simulink model "get_step"  (R2020b)
settings: Solver=FixedStepAuto  StartTime=0.0  StopTime=90  MaxStep=1  RelTol=1e-3
undefined symbols (not defined in the file or in its folder): plant_1
settings Model: Creator=user1  LastModifiedBy=rafael
settings SFSimCC: CustomCodeUndefinedFunction=UseInterfaceOnly

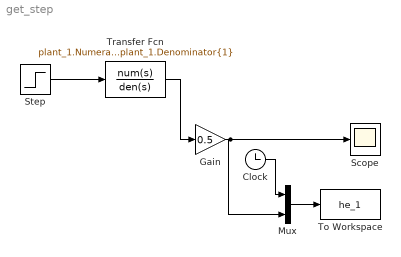
== system get_step ==
  Clock : Clock
  Gain : Gain  Gain=0.5
  Mux : Mux  Inputs=2
  Scope : Scope
  Step : Step  SampleTime=0
  To Workspace : ToWorkspace  VariableName=he_1  SampleTime=-1
      settings: Save2DSignal=2-D array (concatenate along first dimension)
  Transfer Fcn : TransferFcn  Numerator=plant_1.Numerator{1}  Denominator=plant_1.Denominator{1}
  wires:
  Mux/1 -> To Workspace/1
  Clock/1 -> Mux/1
  Step/1 -> Transfer Fcn/1
  Gain/1 -> Mux/2, Scope/1
  Transfer Fcn/1 -> Gain/1
